simulink model "gnc_simplified"  (R2025b)
settings: Solver=ode2  StartTime=0.0  StopTime=inf  FixedStep=1/100  RelTol=1e-3
undefined symbols (not defined in the file or in its folder): DiscIntNeverNeededParam, dspblkCoreblockFVToolHelper, gcbh
libraries: simulink x5, eeGeneralControl x5
(part 1 of 4)
settings Model: Creator=ac112430  LastModifiedBy=ac124458
settings SolverCC: AlgebraicLoopSolver=TrustRegion
settings DataIOCC: ReturnWorkspaceOutputs=off
settings OptimizationCC: DefaultParameterBehavior=Inlined  DefaultUnderspecifiedDataType=single  PassReuseOutputArgsAs=Individual arguments  DifferentSizesBufferReuse=on  EfficientTunableParamExpr=on
settings DebuggingCC: ParameterPrecisionLossMsg=none  ParameterTunabilityLossMsg=error  UnconnectedInputMsg=warning  UnconnectedOutputMsg=warning  UnconnectedLineMsg=warning  BusObjectLabelMismatch=none  ArithmeticOperatorsInVariantConditions=warning
settings HardwareCC: ProdBitPerPointer=32.0  ProdBitPerSizeT=32.0  ProdBitPerPtrDiffT=32.0  ProdLargestAtomicInteger=Long  ProdLargestAtomicFloat=Double  ProdIntDivRoundTo=Undefined  ProdWordSize=32.0  ProdLongLongMode=on  ProdHWDeviceType=ARM Compatible->ARM Cortex
settings ModelReferenceCC: EnableRefExpFcnMdlSchedulingChecks=on  ModelReferenceNumInstancesAllowed=Single  PropagateSignalLabelsOutOfModel=off
settings SFSimCC: SimUseLocalCustomCode=off  MATLABDynamicMemAlloc=off  CustomCodeUndefinedFunction=UseInterfaceOnly
settings RTWCC: SystemTargetFile=ert.tlc  GenCodeOnly=on  TemplateMakefile=ert_default_tmf  RTWUseLocalCustomCode=off  IncludeHyperlinkInReport=on  GPUComputeCapability=3.5  Description=Embedded Coder
settings CodeAppCC: IgnoreCustomStorageClasses=off  MaxIdLength=2048.0  StateflowObjectComments=on
settings ERTTargetCC: ERTCustomFileTemplate=example_file_process.tlc  ConvertIfToSwitch=off  SuppressUnreachableDefaultCases=off  DynamicArrayContainerType=coder::array  TargetLangStandard=C99 (ISO)  GenerateSampleERTMain=on  SupportComplex=off  SupportVariableSizeSignals=on

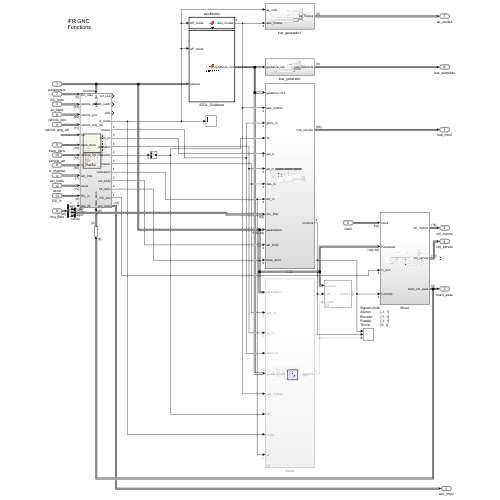
[thumbnail: Simulink's stored preview of the top-level diagram]
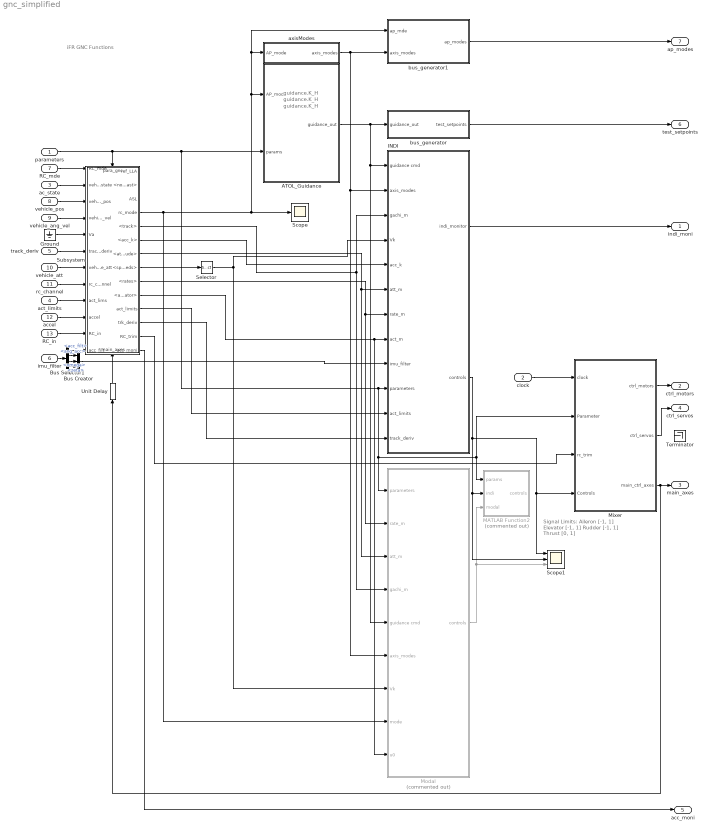
== system gnc_simplified ==
  note: iFR GNC Functions
  note: Signal Limits:
      | Aileron		[-1, 1]
      | Elevator		[-1, 1]
      | Rudder		[-1, 1]
      | Thrust		[0, 1]
  note: guidance.K_H
  note: guidance.K_H
  note: guidance.K_H
  note: guidance.K_H
  note: guidance.K_H
  parameters : Inport  OutDataTypeStr=Bus: IFRCG_Bus_Params_Gnc
  clock : Inport  Port=2  OutDataTypeStr=Bus: IFRCG_Bus_CodeGenInternalClock
  ac_state : Inport  Port=3  OutDataTypeStr=Bus: IFRCG_Bus_Topic_VehicleState  PortDimensions=1  SampleTime=[0.01,0]
  act_limits : Inport  Port=4  OutDataTypeStr=Bus: IFRCG_Bus_Topic_ActuatorLimits
  track_deriv : Inport  Port=5  OutDataTypeStr=Bus: IFRCG_Bus_Topic_TrackDerivMonitor
  imu_filter : Inport  Port=6  OutDataTypeStr=Bus: IFRCG_Bus_Topic_IfrImuFiltered
  RC_mde : Inport  Port=7  OutDataTypeStr=Bus: IFRCG_Bus_Topic_RcMode
  vehicle_pos : Inport  Port=8  OutDataTypeStr=Bus: IFRCG_Bus_Topic_VehicleLocalPosition
  vehicle_ang_vel : Inport  Port=9  OutDataTypeStr=Bus: IFRCG_Bus_Topic_VehicleAngularVelocity
  vehicle_att : Inport  Port=10  OutDataTypeStr=Bus: IFRCG_Bus_Topic_VehicleAttitude
  rc_channel : Inport  Port=11  OutDataTypeStr=Bus: IFRCG_Bus_Topic_RcChannels
  accel : Inport  Port=12  OutDataTypeStr=Bus: IFRCG_Bus_Topic_SensorAccel
  RC_in : Inport  Port=13  OutDataTypeStr=Bus: IFRCG_Bus_Topic_RcTrim
  ATOL_Guidance : MATLAB Function  TreatAsAtomicUnit=on
  Bus Creator : BusCreator  Inputs=3
  Bus Selector1 : BusSelector  OutputSignals=acc_filt,ang_acc,omega,zeta
  Ground : Ground
  INDI : Subsystem
  MATLAB Function2 : MATLAB Function  Commented=on  TreatAsAtomicUnit=on
  Mixer : Subsystem
  Modal : Subsystem  Commented=on
  Scope : Scope
      settings: DataLoggingVariableName=ScopeData4
  Scope1 : Scope  NumInputPorts=3
      settings: ActiveDisplayYMinimum=-1  ActiveDisplayYMaximum=1  DataLoggingVariableName=ScopeData2
  Selector : Selector  InputPortWidth=2  IndexOptions=Index vector (dialog)  Indices=1  OutputSizes=1
  Subsystem : Subsystem
      settings: PortSchema="{\"entries\":[{\"content\":{\"sides\":[{\"content\":{\"connectorIds\":[\"In1\",\"In2\",\"In3\",\"In4\",\"In5\",\"In6\",\"In7\",\"In8\",\"In9\",\"In10\",\"In11\",\"In12\"]},\"type\":\"ConnectorPlacement.EquallySpacedRectSide\",\"uuid\":\"eae11f8f-df23-443f-af8c-32e17e4605f0\"},{\"content\":{\"connectorIds\":[\"Out1\",\"Out2\",\"Out3\",\"Out4\",\"Out5\",\"Out6\",\"Out7\",\"Out8\",\"Out9\",\"Out10\",\"Out11\",\"Out12\",\"Out13\",\"Out14\"],\"side\":\"RIGHT\"},\"type\":\"ConnectorPlacement.EquallySpacedRectSide\",\"uuid\":\"25c6a971-14b0-4ed1-9e4e-a0a3a34e6a3d\"},{\"content\":{\"connectorIds\":[\"In13\"],\"side\":\"TOP\"},\"type\":\"ConnectorPlacement.EquallySpacedRectSide\",\"uuid\":\"38764348-8a10-4184-b281-810ae850f533\"},{\"content\":{\"connectorIds\":[\"In14\"],\"side\":\"BOTTOM\"},\"type\":\"ConnectorPlacement.EquallySpacedRectSide\",\"uuid\":\"a4d29612-f53e-4299-8f37-c5a613e7ffff\"}]},\"type\":\"ConnectorPlacement.EquallySpacedConnector\",\"uuid\":\"9dbe3133-1740-4116-b0d1-43b1503b7370\"}],\"packageUris\":[\"http://schema.mathworks.com/mf0/Connector/R2020b\"],\"version\":\"1.0\"}"
  Terminator : Terminator
  Unit Delay : UnitDelay  SampleTime=-1  HasFrameUpgradeWarning=on
  axisModes : MATLAB Function  TreatAsAtomicUnit=on
  bus_generator : Subsystem
  bus_generator1 : Subsystem
  indi_moni : Outport  OutDataTypeStr=Bus: IFRCG_Bus_Topic_IndiMonitor
  ctrl_motors : Outport  Port=2  OutDataTypeStr=Bus: IFRCG_Bus_Topic_ActuatorMotors  VectorParamsAs1DForOutWhenUnconnected=off
  main_axes : Outport  Port=3  OutDataTypeStr=Bus: IFRCG_Bus_Topic_MainCtrlAxes
  ctrl_servos : Outport  Port=4  OutDataTypeStr=Bus: IFRCG_Bus_Topic_ActuatorServos  VectorParamsAs1DForOutWhenUnconnected=off
  acc_moni : Outport  Port=5  OutDataTypeStr=Bus: IFRCG_Bus_Topic_AccelMonitor
  test_setpoints : Outport  Port=6  OutDataTypeStr=Bus: IFRCG_Bus_Topic_TestSetpointsMonitor
  ap_modes : Outport  Port=7  OutDataTypeStr=Bus: IFRCG_Bus_Topic_ApState
  wires:
  Mixer/1(ctrl_motors) -> ctrl_motors/1
  INDI/1(indi_monitor) -> indi_moni/1
  clock/1 -> Mixer/1(clock)
  ATOL_Guidance/1(guidance_out) -> Modal/5(guidance cmd), INDI/1(guidance cmd), bus_generator/1(guidance_out)
  Subsystem/8(<speeds>) -> Selector/1
  Selector/1 -> Modal/7(Vk), INDI/4(Vk)
  Subsystem/11(act_limits) -> INDI/11(act_limits)
  Subsystem/13(RC_trim) -> Mixer/3(rc_trim)
  Subsystem/6(<acc_k>) -> INDI/5(acc_k)
  Subsystem/7(<attitude>) -> Modal/3(att_m), INDI/6(att_m)
  Subsystem/5(<track>) -> INDI/3(gachi_m), Modal/4(gachi_m)
  ac_state/1 -> Subsystem/2(vehicle_state)
  Subsystem/9(<rates>) -> Modal/2(rate_m), INDI/7(rate_m)
  Subsystem/10(<actuator>) -> Modal/9(u0), INDI/8(act_m)
  Subsystem/12(trk_deriv) -> INDI/12(track_deriv)
  Modal/1(controls) -> Scope1/3, MATLAB Function2/3(modal)
  INDI/2(controls) -> Scope1/1, Mixer/4(Controls), Scope1/2, MATLAB Function2/2(indi)
  axisModes/1(axis_modes) -> Modal/6(axis_modes), INDI/2(axis_modes), bus_generator1/2(axis_modes)
  RC_mde/1 -> Subsystem/1(RC_mde)
  Mixer/3(main_ctrl_axes) -> Unit Delay/1, main_axes/1
  Mixer/2(ctrl_servos) -> ctrl_servos/1
  vehicle_ang_vel/1 -> Subsystem/4(vehicle_ang_vel)
  vehicle_att/1 -> Subsystem/7(vehicle_att)
  vehicle_pos/1 -> Subsystem/3(vehicle_pos)
  Ground/1 -> Subsystem/5(Va)
  act_limits/1 -> Subsystem/9(act_lims)
  Unit Delay/1 -> Subsystem/14(main_axes)
  rc_channel/1 -> Subsystem/8(rc_channel)
  accel/1 -> Subsystem/10(accel)
  imu_filter/1 -> Bus Selector1/1
  Bus Selector1/1 -> Subsystem/12(acc_filt)  "<acc_filt>"
  Bus Selector1/2 -> Bus Creator/1  "<ang_acc>"
  Bus Selector1/3 -> Bus Creator/2  "<omega>"
  Bus Selector1/4 -> Bus Creator/3  "<zeta>"
  Bus Creator/1 -> INDI/9(imu_filter)
  RC_in/1 -> Subsystem/11(RC_in)
  track_deriv/1 -> Subsystem/6(track_deriv)
  Subsystem/14(acc_moni) -> acc_moni/1
  Subsystem/4(rc_mode) -> bus_generator1/1(ap_mde), axisModes/1(AP_mode), ATOL_Guidance/1(AP_mode), Scope/1, Modal/8(mode)
  parameters/1 -> Subsystem/13(para_gnc), Modal/1(parameters), Mixer/2(Parameter), MATLAB Function2/1(params), INDI/10(parameters), ATOL_Guidance/2(params)
  bus_generator/1(test_setpoints) -> test_setpoints/1
  bus_generator1/1(ap_modes) -> ap_modes/1

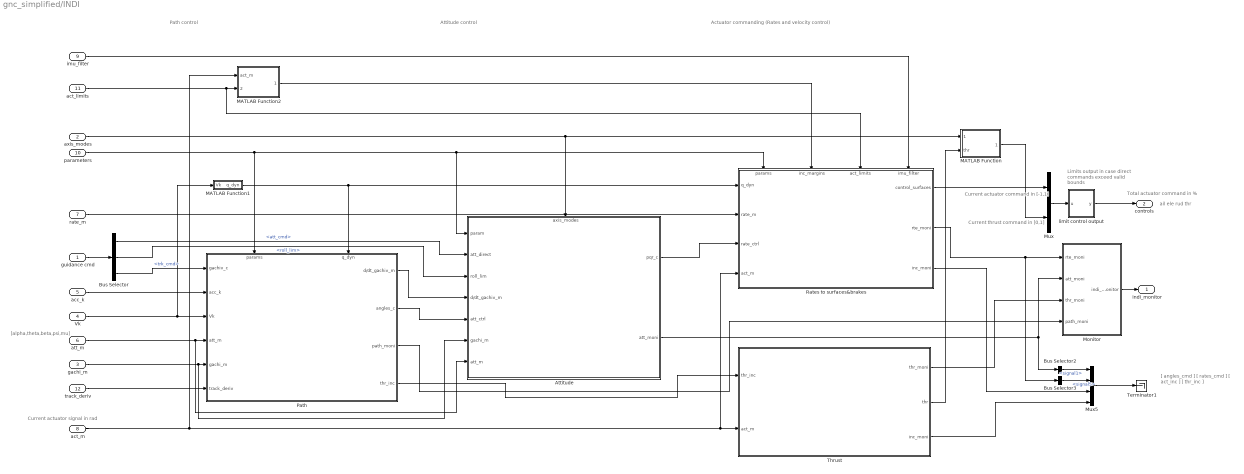
== system gnc_simplified/INDI ==
  note: [ angles_cmd	]
      | [ rates_cmd	]
      | [ act_inc		]
      | [ thr_inc		]
  note: ail ele rud thr
  note: Path control
  note: Current actuator
      | signal in rad
  note: [alpha,theta,beta,psi,mu]
  note: Attitude control
  note: Actuator commanding (Rates and velocity control)
  note: Limits output in case
      | direct commands
      | exceed valid bounds
  note: Current thrust command in [0,1]
  note: Total actuator
      | command in %
  note: Current actuator command in [-1,1]
  guidance cmd : Inport  OutDataTypeStr=Bus: IFRCG_Bus_GuidanceCmd
  axis_modes : Inport  Port=2  OutDataTypeStr=int8
  gachi_m : Inport  Port=3
  Vk : Inport  Port=4  PortDimensions=1
  acc_k : Inport  Port=5
  att_m : Inport  Port=6  OutDataTypeStr=single  PortDimensions=5
  rate_m : Inport  Port=7  OutDataTypeStr=single  PortDimensions=3
  act_m : Inport  Port=8  OutDataTypeStr=single  PortDimensions=4
  imu_filter : Inport  Port=9
  parameters : Inport  Port=10  OutDataTypeStr=Bus: IFRCG_Bus_Params_Gnc
  act_limits : Inport  Port=11
  track_deriv : Inport  Port=12  OutDataTypeStr=single  PortDimensions=2
  Attitude : Subsystem
      settings: PortSchema="{\"entries\":[{\"content\":{\"sides\":[{\"content\":{\"connectorIds\":[\"In1\",\"In2\",\"In3\",\"In4\",\"In5\",\"In6\",\"In7\"]},\"type\":\"ConnectorPlacement.EquallySpacedRectSide\",\"uuid\":\"b7c7e1a9-3024-403b-8101-4fc7eff0575e\"},{\"content\":{\"connectorIds\":[\"Out1\",\"Out2\"],\"side\":\"RIGHT\"},\"type\":\"ConnectorPlacement.EquallySpacedRectSide\",\"uuid\":\"cb53e122-7831-4c34-8aea-2b31ecc7af3b\"},{\"content\":{\"connectorIds\":[\"In8\"],\"side\":\"TOP\"},\"type\":\"ConnectorPlacement.EquallySpacedRectSide\",\"uuid\":\"4b53ef0a-efac-44dd-914a-4d2217d9826d\"}]},\"type\":\"ConnectorPlacement.EquallySpacedConnector\",\"uuid\":\"b88ec9b5-5f11-4970-871c-b4ff42b920b3\"}],\"packageUris\":[\"http://schema.mathworks.com/mf0/Connector/R2020b\"],\"version\":\"1.0\"}"
  Bus Selector : BusSelector  OutputSignals=att_cmd,roll_lim,trk_cmd
  Bus Selector2 : BusSelector  OutputSignals=signal1
  Bus Selector3 : BusSelector  OutputSignals=signal1.signal5
  MATLAB Function : MATLAB Function  TreatAsAtomicUnit=on
  MATLAB Function1 : MATLAB Function  TreatAsAtomicUnit=on
  MATLAB Function2 : MATLAB Function  TreatAsAtomicUnit=on
  Monitor : Subsystem
  Mux : Mux  Inputs=2
  Mux5 : Mux
  Path : Subsystem
      settings: PortSchema="{\"entries\":[{\"content\":{\"sides\":[{\"content\":{\"connectorIds\":[\"In1\",\"In2\",\"In3\",\"In4\",\"In5\",\"In6\"]},\"type\":\"ConnectorPlacement.EquallySpacedRectSide\",\"uuid\":\"aeeb4c65-4157-49e3-89f2-8442de4c35c3\"},{\"content\":{\"connectorIds\":[\"Out1\",\"Out2\",\"Out3\",\"Out4\"],\"side\":\"RIGHT\"},\"type\":\"ConnectorPlacement.EquallySpacedRectSide\",\"uuid\":\"9484377b-093c-4072-8beb-471d4a7ab8a9\"},{\"content\":{\"connectorIds\":[\"In7\",\"In8\"],\"side\":\"TOP\"},\"type\":\"ConnectorPlacement.EquallySpacedRectSide\",\"uuid\":\"c6253d73-40c9-4522-8e2e-6cc388a7bc53\"},{\"content\":{\"side\":\"BOTTOM\"},\"type\":\"ConnectorPlacement.EquallySpacedRectSide\",\"uuid\":\"b5f53673-25a9-4222-bcda-17be59006191\"}]},\"type\":\"ConnectorPlacement.EquallySpacedConnector\",\"uuid\":\"6ddcfaaa-ad15-4bea-bdab-3495e7fd8cf9\"}],\"packageUris\":[\"http://schema.mathworks.com/mf0/Connector/R2020b\"],\"version\":\"1.0\"}"
  Rates to surfaces&brakes : Subsystem
      settings: PortSchema="{\"entries\":[{\"content\":{\"sides\":[{\"content\":{\"connectorIds\":[\"In1\",\"In2\",\"In3\",\"In4\"]},\"type\":\"ConnectorPlacement.EquallySpacedRectSide\",\"uuid\":\"38e84281-7140-4c55-a86a-c71fe3b9f0d7\"},{\"content\":{\"connectorIds\":[\"Out1\",\"Out2\",\"Out3\"],\"side\":\"RIGHT\"},\"type\":\"ConnectorPlacement.EquallySpacedRectSide\",\"uuid\":\"18979a8d-3905-4a49-86c3-949277d06de1\"},{\"content\":{\"connectorIds\":[\"In5\",\"In6\",\"In7\",\"In8\"],\"side\":\"TOP\"},\"type\":\"ConnectorPlacement.EquallySpacedRectSide\",\"uuid\":\"2ae550e8-8587-46c8-a90f-db3ecfdcb8e8\"},{\"content\":{\"side\":\"BOTTOM\"},\"type\":\"ConnectorPlacement.EquallySpacedRectSide\",\"uuid\":\"d561a624-fdf7-40a1-bac0-8ec2b91f5f36\"}]},\"type\":\"ConnectorPlacement.EquallySpacedConnector\",\"uuid\":\"df4b2bf7-ea7e-4f09-bf8e-e1a831543136\"}],\"packageUris\":[\"http://schema.mathworks.com/mf0/Connector/R2020b\"],\"version\":\"1.0\"}"
  Terminator1 : Terminator
  Thrust : Subsystem
  limit control output : MATLAB Function  TreatAsAtomicUnit=on
  indi_monitor : Outport  OutDataTypeStr=Bus: IFRCG_Bus_Topic_IndiMonitor
  controls : Outport  Port=2  OutDataTypeStr=single  PortDimensions=4  VectorParamsAs1DForOutWhenUnconnected=off
  wires:
  Bus Selector/2 -> Attitude/3(roll_lim)  "<roll_lim>"
  Thrust/3(inc_moni) -> Mux5/4
  Path/3(path_moni) -> Monitor/4(path_moni)
  Rates to surfaces&brakes/3(inc_moni) -> Mux5/3
  parameters/1 -> Rates to surfaces&brakes/5(params), Attitude/1(param), Path/7(params)
  Mux5/1 -> Terminator1/1
  att_m/1 -> Attitude/7(att_m), Path/4(att_m)
  acc_k/1 -> Path/2(acc_k)
  Rates to surfaces&brakes/1(control_surfaces) -> Mux/1
  Bus Selector/3 -> Path/1(gachiv_c)  "<trk_cmd>"
  Attitude/1(pqr_c) -> Rates to surfaces&brakes/3(rate_ctrl)
  Vk/1 -> MATLAB Function1/1(Vk), Path/3(Vk)
  act_m/1 -> Thrust/2(act_m), Rates to surfaces&brakes/4(act_m), MATLAB Function2/1(act_m)
  Path/4(thr_inc) -> Thrust/1(thr_inc)
  rate_m/1 -> Rates to surfaces&brakes/2(rate_m)
  Path/2(angles_c) -> Attitude/5(att_ctrl)
  Thrust/2(thr) -> MATLAB Function/2(thr)
  guidance cmd/1 -> Bus Selector/1
  Path/1(d/dt_gachiv_m) -> Attitude/4(d/dt_gachiv_m)
  Thrust/1(thr_moni) -> Monitor/3(thr_moni)
  Rates to surfaces&brakes/2(rte_moni) -> Monitor/1(rte_moni), Bus Selector3/1
  gachi_m/1 -> Attitude/6(gachi_m), Path/5(gachi_m)
  Monitor/1(indi_monitor) -> indi_monitor/1
  Bus Selector2/1 -> Mux5/1  "<signal1>"
  Bus Selector3/1 -> Mux5/2  "<signal5>"
  Attitude/2(att_moni) -> Monitor/2(att_moni), Bus Selector2/1
  track_deriv/1 -> Path/6(track_deriv)
  limit control output/1(y) -> controls/1
  act_limits/1 -> Rates to surfaces&brakes/7(act_limits), MATLAB Function2/2(act_limit)
  MATLAB Function2/1(inc_margins) -> Rates to surfaces&brakes/6(inc_margins)
  imu_filter/1 -> Rates to surfaces&brakes/8(imu_filter)
  Mux/1 -> limit control output/1(u)
  axis_modes/1 -> MATLAB Function/1(axis_modes), Attitude/8(axis_modes)
  MATLAB Function/1(thr_cmd) -> Mux/2
  Bus Selector/1 -> Attitude/2(att_direct)  "<att_cmd>"
  MATLAB Function1/1(q_dyn) -> Rates to surfaces&brakes/1(q_dyn), Path/8(q_dyn)

== system gnc_simplified/Mixer ==
  note: control allocation for elevator and rudder
  note: Reversing ap output according to servo mounting direction;
  note: Adjusting output
      | according to servo
      | limitations
  note: Sorting for channel
      | scaling in Pixhawk
  note: thr
      | ail
      | ele
      | rud
  note: Output for Gram:
      | 1 Thrust
      | 2 Aileron right
      | 3 Aileron left
      | 4 Flaperon right
      | 5 Flaperon left
      | 6 Elevator/Rudder right
      | 7 Elevator/Rudder left
      | 8 Gear
      | 9 Safety
      | 10 Arming
      | 11 Mode switch
  note: Signal Limits:
      | Aileron		[-1, 1]
      | Elevator		[-1, 1]
      | Rudder		[-1, 1]
      | Thrust		[0, 1]
  note: Signal Limits:
      | Aileron		[-1, 1]
      | Elevator		[-1, 1]
      | Rudder		[-1, 1]
      | Thrust		[0, 1]
  clock : Inport  OutDataTypeStr=Bus: IFRCG_Bus_CodeGenInternalClock
  Parameter : Inport  Port=2  OutDataTypeStr=Bus: IFRCG_Bus_Params_Gnc
  rc_trim : Inport  Port=3
  Controls : Inport  Port=4  OutDataTypeStr=single  PortDimensions=4
  Bus Selector : BusSelector  OutputSignals=sys_time_us
  Constant2 : Constant  Value=zeros(8,1)  OutDataTypeStr=single
  Data Type Conversion1 : DataTypeConversion  OutDataTypeStr=uint64  SaturateOnIntegerOverflow=off  RndMeth=Floor
  MATLAB Function1 : MATLAB Function  TreatAsAtomicUnit=on
  MATLAB Function2 : MATLAB Function  TreatAsAtomicUnit=on
  PWM Limiter : MATLAB Function  TreatAsAtomicUnit=on
  Scope1 : Scope  NumInputPorts=2
      settings: ActiveDisplayYMinimum=-1.25  ActiveDisplayYMaximum=1.25  DataLoggingVariableName=ScopeData8
  Scope2 : Scope
      settings: ActiveDisplayYMinimum=-2.2855338454246521  ActiveDisplayYMaximum=2.2855338454246521  DataLoggingVariableName=ScopeData2
  Selector1 : Selector  InputPortWidth=4  IndexOptions=Index vector (dialog)  Indices=[4 1 2 3]  OutputSizes=1
  Terminator : Terminator
  _bus_creator1 : Subsystem
  _bus_creator2 : Subsystem  Commented=on
  bus_generator : Subsystem
  scale_RC_thr : MATLAB Function  TreatAsAtomicUnit=on
  scale_thr : MATLAB Function  TreatAsAtomicUnit=on
  ctrl_motors : Outport  OutDataTypeStr=Bus: IFRCG_Bus_Topic_ActuatorMotors  VectorParamsAs1DForOutWhenUnconnected=off
  ctrl_servos : Outport  Port=2  OutDataTypeStr=Bus: IFRCG_Bus_Topic_ActuatorServos  VectorParamsAs1DForOutWhenUnconnected=off
  main_ctrl_axes : Outport  Port=3  OutDataTypeStr=Bus: IFRCG_Bus_Topic_MainCtrlAxes
  wires:
  Controls/1 -> scale_thr/1(in)  "ail ele rud thr nw"
  Parameter/1 -> PWM Limiter/1(parameter), MATLAB Function1/1(params)
  clock/1 -> Bus Selector/1
  rc_trim/1 -> scale_RC_thr/1(in)
  _bus_creator2/1(actuator_controls) -> Terminator/1
  Constant2/1 -> _bus_creator2/1(control)
  scale_RC_thr/1(out) -> MATLAB Function1/3(rc_controls)
  Selector1/1 -> bus_generator/1(In1), Scope1/2, MATLAB Function2/1(controls_in)
  scale_thr/1(out) -> MATLAB Function1/2(ap_controls), Scope1/1
  MATLAB Function2/1(controls_out) -> PWM Limiter/2(controls)
  _bus_creator1/2(ctrl_servos) -> ctrl_servos/1
  bus_generator/1(main_ctrl_axes) -> main_ctrl_axes/1
  PWM Limiter/1(controlsLtd) -> _bus_creator1/1(control), Scope2/1
  Data Type Conversion1/1 -> _bus_creator1/2(timestamp_sample)
  Bus Selector/1 -> Data Type Conversion1/1, _bus_creator2/2(timestamp_sample)  "<sys_time_us>"
  _bus_creator1/1(ctrl_motors) -> ctrl_motors/1
  MATLAB Function1/1(controls) -> Selector1/1

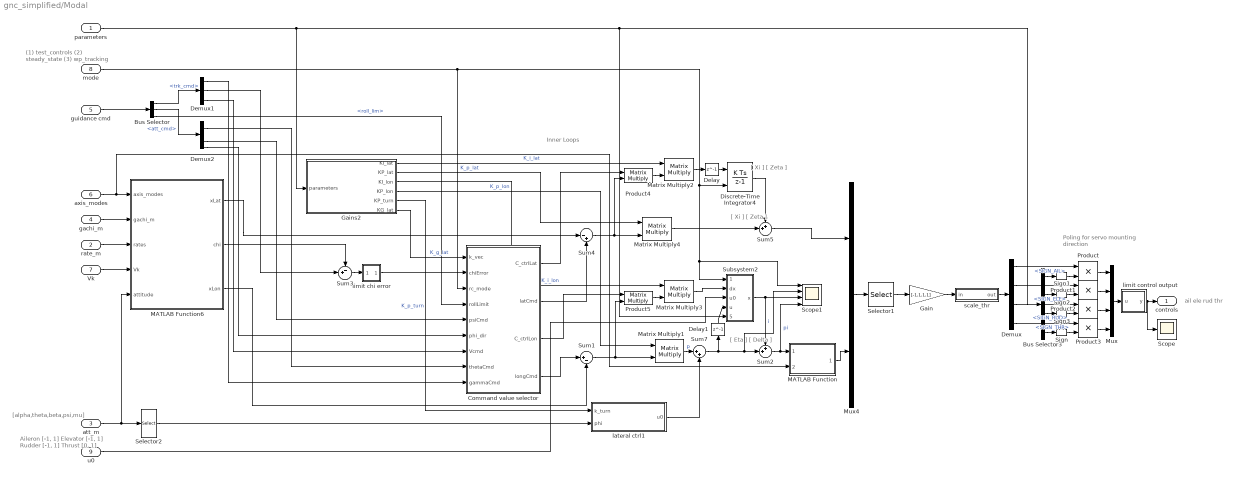
== system gnc_simplified/Modal ==
  note: [alpha,theta,beta,psi,mu]
  note: ail ele rud thr
  note: Poling for servo
      | mounting direction
  note: [ Xi     ]
      | [ Zeta ]
  note: Inner Loops
  note: [ Xi     ]
      | [ Zeta ]
  note: [ Eta    ]
      | [ Delta ]
  note: (1) test_controls
      | (2) steady_state
      | (3) wp_tracking
  note: Aileron		[-1, 1]
      | Elevator		[-1, 1]
      | Rudder		[-1, 1]
      | Thrust		[0, 1]
  parameters : Inport  OutDataTypeStr=Bus: IFRCG_Bus_Params_Gnc
  rate_m : Inport  Port=2  OutDataTypeStr=single  PortDimensions=3
  att_m : Inport  Port=3  OutDataTypeStr=single  PortDimensions=5
  gachi_m : Inport  Port=4
  guidance cmd : Inport  Port=5  OutDataTypeStr=Bus: IFRCG_Bus_GuidanceCmd
  axis_modes : Inport  Port=6
  Vk : Inport  Port=7  PortDimensions=1
  mode : Inport  Port=8  OutDataTypeStr=uint8
  u0 : Inport  Port=9  OutDataTypeStr=single  PortDimensions=4
  Bus Selector : BusSelector  OutputSignals=trk_cmd,att_cmd,roll_lim
  Bus Selector3 : BusSelector  OutputSignals=Ifr_Gnc.SIGN_AIL,Ifr_Gnc.SIGN_ELE,Ifr_Gnc.SIGN_RUD,Ifr_Gnc.SIGN_THR
  Command value selector : MATLAB Function  TreatAsAtomicUnit=on
  Delay : Delay  DelayLength=1
  Delay1 : Delay  DelayLength=1
  Demux : Demux
  Demux1 : Demux  Outputs=3
  Demux2 : Demux  Outputs=5
  Discrete-Time Integrator4 : DiscreteIntegrator  ExternalReset=either  SampleTime=-1  LimitOutput=on  UpperSaturationLimit=15  LowerSaturationLimit=-15  ICPrevOutput=DiscIntNeverNeededParam  ICPrevScaledInput=DiscIntNeverNeededParam
  Gain : Gain  Gain=[-1,1,1,1]
  Gains2 : MATLAB Function  TreatAsAtomicUnit=on
  MATLAB Function : MATLAB Function  TreatAsAtomicUnit=on
  MATLAB Function6 : MATLAB Function  TreatAsAtomicUnit=on
  Matrix Multiply{1..4} (4 alike) : Product  Multiplication=Matrix(*)
  Mux : Mux
  Mux4 : Mux  Inputs=2
  Product{,1..3} (4 alike) : Product  OutDataTypeStr=single
  Product4 : Product  Multiplication=Matrix(*)
  Product5 : Product  Multiplication=Matrix(*)
  Scope : Scope
      settings: DataLoggingVariableName=ScopeData9
  Scope1 : Scope  NumInputPorts=4
      settings: DataLoggingVariableName=ScopeData10
  Selector1 : Selector  InputPortWidth=4  IndexOptions=Index vector (dialog)  Indices=[1,3,2,4]  OutputSizes=1
  Selector2 : Selector  InputPortWidth=5  IndexOptions=Index vector (dialog)  Indices=5  OutputSizes=1
  Sign{,1..3} (4 alike) : Signum
  Subsystem2 : Subsystem
      mask Display:
      | disp('\bf\fontsize{12}\int dx', 'texmode', 'on')
      | port_label('input', 2, 'dx', 'texmode', 'on')
      | port_label('input', 1, 'Tr')
      | port_label('input', 3, 'u_0', 'texmode', 'on')
      | port_label('input', 4, 'u_P', 'texmode', 'on')
      | 
      | port_label('output', 1, 'x', 'texmode', 'on')
  Sum1 : Sum  Inputs=|+-
  Sum2 : Sum  Inputs=++|
  Sum3 : Sum  Inputs=-+|
  Sum4 : Sum  Inputs=|-+
  Sum5 : Sum  Inputs=++|
  Sum7 : Sum  Inputs=|++
  lateral ctrl1 : MATLAB Function  TreatAsAtomicUnit=on
  limit chi error : MATLAB Function  TreatAsAtomicUnit=on
  limit control output : MATLAB Function  TreatAsAtomicUnit=on
  scale_thr : MATLAB Function  TreatAsAtomicUnit=on
  controls : Outport  OutDataTypeStr=single  PortDimensions=4  VectorParamsAs1DForOutWhenUnconnected=off
  wires:
  limit control output/1(y) -> Scope/1, controls/1
  guidance cmd/1 -> Bus Selector/1
  Gain/1 -> scale_thr/1(in)
  Mux4/1 -> Selector1/1
  Selector1/1 -> Gain/1
  Bus Selector/1 -> Demux1/1  "<trk_cmd>"
  Demux/4 -> Product3/1
  Demux/2 -> Product1/1
  Bus Selector3/3 -> Sign3/1  "<SIGN_RUD>"
  Sign/1 -> Product3/2
  Bus Selector3/1 -> Sign1/1  "<SIGN_AIL>"
  Demux/1 -> Product/1
  Bus Selector3/2 -> Sign2/1  "<SIGN_ELE>"
  Sign1/1 -> Product/2
  Demux/3 -> Product2/1
  Bus Selector3/4 -> Sign/1  "<SIGN_THR>"
  Sign2/1 -> Product1/2
  Sign3/1 -> Product2/2
  Product/1 -> Mux/1
  Product1/1 -> Mux/2
  Product2/1 -> Mux/3
  Product3/1 -> Mux/4
  Mux/1 -> limit control output/1(u)
  scale_thr/1(out) -> Demux/1
  MATLAB Function/1(ele_thr_cmd) -> Mux4/2
  Bus Selector/2 -> Demux2/1  "<att_cmd>"
  parameters/1 -> Gains2/1(parameters), Bus Selector3/1, Subsystem2/5(param)
  Sum5/1 -> Mux4/1
  Delay1/1 -> Subsystem2/4(u)
  Delay/1 -> Discrete-Time Integrator4/1
  Command value selector/1(C_ctrlLat) -> Product4/1
  Demux2/4 -> Command value selector/5(psiCmd)
  Gains2/5(KP_turn) -> lateral ctrl1/1(k_turn)  "K_p_turn"
  Product4/1 -> Matrix Multiply2/2
  Gains2/1(KI_lat) -> Matrix Multiply2/1  "K_i_lat"
  Gains2/3(KI_lon) -> Matrix Multiply3/1  "K_i_lon"
  Matrix Multiply1/1 -> Sum7/1  "p"
  Command value selector/2(latCmd) -> Sum4/2
  Gains2/2(KP_lat) -> Matrix Multiply4/1  "K_p_lat"
  Demux1/3 -> Command value selector/7(Vcmd)
  limit chi error/1(y) -> Command value selector/2(chiError)
  Product5/1 -> Matrix Multiply3/2
  Command value selector/4(longCmd) -> Sum1/1
  Demux2/2 -> Command value selector/8(thetaCmd)
  Matrix Multiply3/1 -> Subsystem2/2(dx)
  Command value selector/3(C_ctrlLon) -> Product5/1
  Discrete-Time Integrator4/1 -> Sum5/1
  Demux1/1 -> Command value selector/9(gammaCmd)
  Gains2/4(KP_lon) -> Matrix Multiply1/1  "K_p_lon"
  Subsystem2/1(x) -> Sum2/1, Scope1/3  "i"
  Matrix Multiply2/1 -> Delay/1
  MATLAB Function6/3(xLon) -> Sum1/2
  Sum4/1 -> Product4/2, Matrix Multiply4/2
  lateral ctrl1/1(u0) -> Sum7/2
  MATLAB Function6/1(xLat) -> Sum4/1
  Sum2/1 -> Scope1/4, MATLAB Function/1(ele_thr)  "pi"
  Selector2/1 -> lateral ctrl1/2(phi)
  Bus Selector/3 -> Command value selector/4(rollLimit)  "<roll_lim>"
  u0/1 -> Subsystem2/3(u0)
  Sum3/1 -> limit chi error/1(u)
  Sum1/1 -> Product5/2, Matrix Multiply1/2
  mode/1 -> Discrete-Time Integrator4/2, Scope1/1, Subsystem2/1(mode), Command value selector/3(rc_mode)
  Sum7/1 -> Delay1/1, Scope1/2, Sum2/2
  Matrix Multiply4/1 -> Sum5/2
  MATLAB Function6/2(chi) -> Sum3/1
  att_m/1 -> MATLAB Function6/5(attitude), Selector2/1
  Vk/1 -> MATLAB Function6/4(Vk)
  gachi_m/1 -> MATLAB Function6/2(gachi_m)
  rate_m/1 -> MATLAB Function6/3(rates)
  Demux1/2 -> Sum3/2
  Demux2/5 -> Command value selector/6(phi_dir)
  Gains2/6(KG_lat) -> Command value selector/1(k_vec)  "K_g_lat"
  axis_modes/1 -> MATLAB Function/2(axis_modes), MATLAB Function6/1(axis_modes)

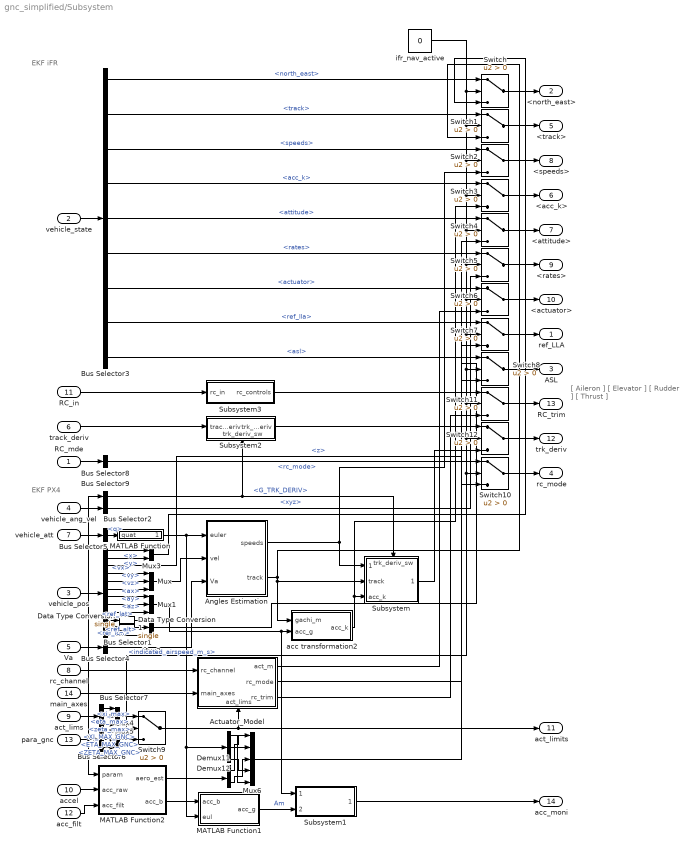
== system gnc_simplified/Subsystem ==
  note: EKF iFR
  note: EKF PX4
  note: [ Aileron	  ]
      | [ Elevator ]
      | [ Rudder	  ]
      | [ Thrust	  ]
  RC_mde : Inport  OutDataTypeStr=Bus: IFRCG_Bus_Topic_RcMode
  vehicle_state : Inport  Port=2  OutDataTypeStr=Bus: IFRCG_Bus_Topic_VehicleState
  vehicle_pos : Inport  Port=3  OutDataTypeStr=Bus: IFRCG_Bus_Topic_VehicleLocalPosition
  vehicle_ang_vel : Inport  Port=4  OutDataTypeStr=Bus: IFRCG_Bus_Topic_VehicleAngularVelocity
  Va : Inport  Port=5  OutDataTypeStr=Bus: IFRCG_Bus_Topic_Airspeed
  track_deriv : Inport  Port=6  OutDataTypeStr=Bus: IFRCG_Bus_Topic_TrackDerivMonitor
  vehicle_att : Inport  Port=7  OutDataTypeStr=Bus: IFRCG_Bus_Topic_VehicleAttitude
  rc_channel : Inport  Port=8  OutDataTypeStr=Bus: IFRCG_Bus_Topic_RcChannels
  act_lims : Inport  Port=9  OutDataTypeStr=Bus: IFRCG_Bus_Topic_ActuatorLimits
  accel : Inport  Port=10  OutDataTypeStr=Bus: IFRCG_Bus_Topic_SensorAccel
  RC_in : Inport  Port=11  OutDataTypeStr=Bus: IFRCG_Bus_Topic_RcTrim
  acc_filt : Inport  Port=12
  para_gnc : Inport  Port=13  OutDataTypeStr=Bus: IFRCG_Bus_Params_Gnc
  main_axes : Inport  Port=14  OutDataTypeStr=Bus: IFRCG_Bus_Topic_MainCtrlAxes
  Actuator_Model : Subsystem
      settings: PortSchema="{\"entries\":[{\"content\":{\"sides\":[{\"content\":{\"connectorIds\":[\"In1\",\"In2\"]},\"type\":\"ConnectorPlacement.EquallySpacedRectSide\",\"uuid\":\"0b560cb0-425b-4e75-ad69-9f3dd2ae247d\"},{\"content\":{\"connectorIds\":[\"Out1\",\"Out2\",\"Out3\"],\"side\":\"RIGHT\"},\"type\":\"ConnectorPlacement.EquallySpacedRectSide\",\"uuid\":\"67043da2-be34-4466-be37-15cebe548400\"},{\"content\":{\"side\":\"TOP\"},\"type\":\"ConnectorPlacement.EquallySpacedRectSide\",\"uuid\":\"dbc9e13d-738a-4a6f-867f-431ba88297cf\"},{\"content\":{\"connectorIds\":[\"In3\"],\"side\":\"BOTTOM\"},\"type\":\"ConnectorPlacement.EquallySpacedRectSide\",\"uuid\":\"14b82ace-20eb-4480-853b-ffa5dbbc5ee0\"}]},\"type\":\"ConnectorPlacement.EquallySpacedConnector\",\"uuid\":\"43045ae4-5565-43c8-8df8-998e069be6cd\"}],\"packageUris\":[\"http://schema.mathworks.com/mf0/Connector/R2020b\"],\"version\":\"1.0\"}"
  Angles Estimation : MATLAB Function  TreatAsAtomicUnit=on
  Bus Selector1 : BusSelector  OutputSignals=x,y,z,vx,vy,vz,ax,ay,az,ref_lat,ref_lon,ref_alt
  Bus Selector2 : BusSelector  OutputSignals=xyz
  Bus Selector3 : BusSelector  OutputSignals=north_east,track,speeds,acc_k,attitude,rates,actuator,ref_lla,asl
  Bus Selector4 : BusSelector  OutputSignals=indicated_airspeed_m_s
  Bus Selector5 : BusSelector  OutputSignals=q
  Bus Selector6 : BusSelector  OutputSignals=Ifr_Gnc.XI_MAX_GNC,Ifr_Gnc.ETA_MAX_GNC,Ifr_Gnc.ZETA_MAX_GNC
  Bus Selector7 : BusSelector  OutputSignals=xi_max,eta_max,zeta_max
  Bus Selector8 : BusSelector  OutputSignals=rc_mode
  Bus Selector9 : BusSelector  OutputSignals=Ifr_Gnc.G_TRK_DERIV
  Data Type Conversion : DataTypeConversion  OutDataTypeStr=single  SaturateOnIntegerOverflow=off  RndMeth=Floor
  Data Type Conversion1 : DataTypeConversion  OutDataTypeStr=single  SaturateOnIntegerOverflow=off  RndMeth=Floor
  Demux11 : Demux  Outputs=2
  Demux12 : Demux  Outputs=3
  MATLAB Function : MATLAB Function  TreatAsAtomicUnit=on
  MATLAB Function1 : MATLAB Function  TreatAsAtomicUnit=on
  MATLAB Function2 : MATLAB Function  TreatAsAtomicUnit=on
  Mux{,1..2,4..5} (5 alike) : Mux  Inputs=3
  Mux3 : Mux  Inputs=2
  Mux6 : Mux  Inputs=5
  Subsystem : Subsystem
      settings: PortSchema="{\"entries\":[{\"content\":{\"sides\":[{\"content\":{\"connectorIds\":[\"In1\",\"In2\",\"In3\"]},\"type\":\"ConnectorPlacement.EquallySpacedRectSide\",\"uuid\":\"d3f70b0d-5808-41a1-901a-3e2b7a37eb93\"},{\"content\":{\"connectorIds\":[\"Out1\"],\"side\":\"RIGHT\"},\"type\":\"ConnectorPlacement.EquallySpacedRectSide\",\"uuid\":\"dc4ca20c-eb1b-4454-88d2-269a48f937e4\"},{\"content\":{\"connectorIds\":[\"In4\"],\"side\":\"TOP\"},\"type\":\"ConnectorPlacement.EquallySpacedRectSide\",\"uuid\":\"1dace743-43be-4004-9081-e38a97e7a582\"}]},\"type\":\"ConnectorPlacement.EquallySpacedConnector\",\"uuid\":\"5771c896-d5ee-401f-a70a-0ba475a64d58\"}],\"packageUris\":[\"http://schema.mathworks.com/mf0/Connector/R2020b\"],\"version\":\"1.0\"}"
  Subsystem1 : Subsystem
  Subsystem2 : Subsystem
      settings: PortSchema="{\"entries\":[{\"content\":{\"sides\":[{\"content\":{\"connectorIds\":[\"In1\"]},\"type\":\"ConnectorPlacement.EquallySpacedRectSide\",\"uuid\":\"c249bde2-4580-435b-8669-29d5f206d176\"},{\"content\":{\"connectorIds\":[\"Out1\"],\"side\":\"RIGHT\"},\"type\":\"ConnectorPlacement.EquallySpacedRectSide\",\"uuid\":\"60962190-2f64-42e9-bf1a-6d4a20eea6b3\"},{\"content\":{\"side\":\"TOP\"},\"type\":\"ConnectorPlacement.EquallySpacedRectSide\",\"uuid\":\"d4f64458-133b-4324-95a6-14c38555dd9a\"},{\"content\":{\"connectorIds\":[\"In2\"],\"side\":\"BOTTOM\"},\"type\":\"ConnectorPlacement.EquallySpacedRectSide\",\"uuid\":\"5ed7f531-edd6-4543-875a-2dd5af02d360\"}]},\"type\":\"ConnectorPlacement.EquallySpacedConnector\",\"uuid\":\"8eaaea99-2870-4f7f-ab6c-9598fb8c4fc7\"}],\"packageUris\":[\"http://schema.mathworks.com/mf0/Connector/R2020b\"],\"version\":\"1.0\"}"
  Subsystem3 : Subsystem
  Switch{,1..12} (13 alike) : Switch  Criteria=u2 > Threshold  SaturateOnIntegerOverflow=off  InputSameDT=off
  acc transformation2 : MATLAB Function  TreatAsAtomicUnit=on
  ifr_nav_active : Constant  Value=0
  ref_LLA : Outport
  <north_east> : Outport  Port=2
  ASL : Outport  Port=3
  rc_mode : Outport  Port=4  OutDataTypeStr=uint8  PortDimensions=1
  <track> : Outport  Port=5
  <acc_k> : Outport  Port=6
  <attitude> : Outport  Port=7
  <speeds> : Outport  Port=8
  <rates> : Outport  Port=9
  <actuator> : Outport  Port=10
  act_limits : Outport  Port=11
  trk_deriv : Outport  Port=12  PortDimensions=2
  RC_trim : Outport  Port=13  PortDimensions=4
  acc_moni : Outport  Port=14  OutDataTypeStr=Bus: IFRCG_Bus_Topic_AccelMonitor
  wires:
  Bus Selector3/5 -> Switch4/1  "<attitude>"
  Bus Selector3/4 -> Switch3/1  "<acc_k>"
  Bus Selector3/7 -> Switch6/1  "<actuator>"
  Bus Selector3/1 -> Switch/1  "<north_east>"
  Bus Selector3/2 -> Switch1/1  "<track>"
  Bus Selector3/6 -> Switch5/1  "<rates>"
  Bus Selector3/3 -> Switch2/1  "<speeds>"
  vehicle_state/1 -> Bus Selector3/1
  Bus Selector2/1 -> Switch5/3  "<xyz>"
  Angles Estimation/2(track) -> Subsystem/2(track), acc transformation2/1(gachi_m), Switch1/3
  vehicle_att/1 -> Bus Selector5/1
  Bus Selector5/1 -> MATLAB Function/1(quat)  "<q>"
  Bus Selector1/2 -> Mux3/2  "<y>"
  vehicle_ang_vel/1 -> Bus Selector2/1
  Bus Selector4/1 -> Angles Estimation/3(Va)  "<indicated_airspeed_m_s>"
  Bus Selector1/5 -> Mux/2  "<vy>"
  Va/1 -> Bus Selector4/1
  Bus Selector1/4 -> Mux/1  "<vx>"
  vehicle_pos/1 -> Bus Selector1/1
  Bus Selector1/6 -> Mux/3  "<vz>"
  Mux/1 -> Angles Estimation/2(vel)
  Bus Selector1/1 -> Mux3/1  "<x>"
  Bus Selector1/7 -> Mux1/1  "<ax>"
  Bus Selector1/8 -> Mux1/2  "<ay>"
  Bus Selector1/9 -> Mux1/3  "<az>"
  Mux1/1 -> Subsystem1/1(acc_g_vlp), acc transformation2/2(acc_g)
  acc transformation2/1(acc_k) -> Switch3/3, Subsystem/3(acc_k)
  MATLAB Function/1(eul_rad) -> Angles Estimation/1(euler), MATLAB Function1/2(eul), Demux12/1
  Angles Estimation/1(speeds) -> Subsystem/1(speeds), Switch2/3
  Mux3/1 -> Switch/3
  Bus Selector3/8 -> Switch7/1  "<ref_lla>"
  Bus Selector3/9 -> Switch8/1  "<asl>"
  Switch/1 -> <north_east>/1
  Switch1/1 -> <track>/1
  Switch2/1 -> <speeds>/1
  Switch3/1 -> <acc_k>/1
  Switch4/1 -> <attitude>/1
  Switch5/1 -> <rates>/1
  Switch8/1 -> ASL/1
  Switch6/1 -> <actuator>/1
  Switch7/1 -> ref_LLA/1
  Actuator_Model/1(act_m) -> Switch6/3
  Bus Selector1/10 -> Data Type Conversion/1  "<ref_lat>"
  Bus Selector1/11 -> Data Type Conversion1/1  "<ref_lon>"
  Bus Selector1/12 -> Mux2/3  "<ref_alt>"
  Bus Selector1/3 -> Switch8/3  "<z>"
  rc_channel/1 -> Actuator_Model/1(rc_channel)
  main_axes/1 -> Actuator_Model/2(main_axes)
  act_lims/1 -> Bus Selector7/1
  Switch9/1 -> Actuator_Model/3(act_lims), act_limits/1
  ifr_nav_active/1 -> Switch/2, Switch1/2, Switch2/2, Switch3/2, Switch4/2, Switch5/2, Switch6/2, Switch7/2, Switch11/2, Switch12/2, Switch9/2, Switch10/2, Switch8/2
  para_gnc/1 -> MATLAB Function2/1(param), Bus Selector9/1, Bus Selector6/1
  Mux4/1 -> Switch9/3
  Bus Selector6/1 -> Mux4/1  "<XI_MAX_GNC>"
  Bus Selector6/2 -> Mux4/2  "<ETA_MAX_GNC>"
  Bus Selector6/3 -> Mux4/3  "<ZETA_MAX_GNC>"
  Bus Selector7/1 -> Mux5/1  "<xi_max>"
  Bus Selector7/2 -> Mux5/2  "<eta_max>"
  Bus Selector7/3 -> Mux5/3  "<zeta_max>"
  Mux5/1 -> Switch9/1
  Actuator_Model/2(rc_mode) -> Switch10/3
  RC_mde/1 -> Bus Selector8/1
  Switch10/1 -> rc_mode/1
  Demux12/1 -> Mux6/5
  Demux11/2 -> Mux6/3
  Demux11/1 -> Mux6/1
  Demux12/3 -> Mux6/4
  Demux12/2 -> Mux6/2
  Mux6/1 -> Switch4/3
  MATLAB Function2/1(aero_est) -> Demux11/1
  accel/1 -> MATLAB Function2/2(acc_raw)
  acc_filt/1 -> MATLAB Function2/3(acc_filt)
  Bus Selector8/1 -> Switch10/1  "<rc_mode>"
  Mux2/1 -> Switch7/3
  Data Type Conversion/1 -> Mux2/1
  Data Type Conversion1/1 -> Mux2/2
  Actuator_Model/3(rc_trim) -> Switch11/3
  Switch11/1 -> RC_trim/1
  Subsystem3/1(rc_controls) -> Switch11/1
  Switch12/1 -> trk_deriv/1
  Subsystem2/1(trk_deriv) -> Switch12/1
  Subsystem/1(d_trk_moni) -> Switch12/3
  MATLAB Function2/2(acc_b) -> MATLAB Function1/1(acc_b)
  MATLAB Function1/1(acc_g) -> Subsystem1/2(acc_g_filt)  "Am"
  Subsystem1/1(acc_moni) -> acc_moni/1
  track_deriv/1 -> Subsystem2/1(track_deriv)
  RC_in/1 -> Subsystem3/1(rc_in)
  Bus Selector9/1 -> Subsystem2/2(trk_deriv_sw), Subsystem/4(trk_deriv_sw)  "<G_TRK_DERIV>"

== system gnc_simplified/bus_generator ==
  guidance_out : Inport  OutDataTypeStr=Bus: IFRCG_Bus_GuidanceCmd
  Bus Creator : BusCreator  Inputs=8  OutDataTypeStr=Bus: IFRCG_Bus_Topic_TestSetpointsMonitor
      settings: InheritFromInputs=off
  Bus Selector : BusSelector  OutputSignals=trk_cmd,att_cmd
  Demux : Demux  Outputs=2
  Demux1 : Demux  Outputs=3
  Selector : Selector  InputPortWidth=3  IndexOptions=Index vector (dialog)  Indices=[1 3]  OutputSizes=1
  Selector1 : Selector  InputPortWidth=5  IndexOptions=Index vector (dialog)  Indices=[5 2 4]  OutputSizes=1
  codegen_topic_publication : Subsystem
  codegen_topic_subscription : Subsystem
  publish_topic : Constant  Value=true  OutDataTypeStr=boolean
  timestamp : Constant  Value=0  OutDataTypeStr=uint64
  test_setpoints : Outport  OutDataTypeStr=Bus: IFRCG_Bus_Topic_TestSetpointsMonitor
  wires:
  Demux1/3 -> Bus Creator/6
  Demux/2 -> Bus Creator/3
  Bus Creator/1 -> test_setpoints/1
  timestamp/1 -> Bus Creator/1
  Demux1/1 -> Bus Creator/4
  publish_topic/1 -> codegen_topic_publication/1(publish_topic)
  codegen_topic_publication/1(bus_codegen_topic_publication) -> Bus Creator/8
  codegen_topic_subscription/1(bus_codegen_topic_subscription) -> Bus Creator/7
  guidance_out/1 -> Bus Selector/1
  Demux1/2 -> Bus Creator/5
  Demux/1 -> Bus Creator/2
  Bus Selector/2 -> Selector1/1  "<att_cmd>"
  Bus Selector/1 -> Selector/1  "<trk_cmd>"
  Selector/1 -> Demux/1
  Selector1/1 -> Demux1/1

== system gnc_simplified/bus_generator1 ==
  ap_mde : Inport  OutDataTypeStr=uint8
  axis_modes : Inport  Port=2
  Bus Creator : BusCreator  Inputs=8  OutDataTypeStr=Bus: IFRCG_Bus_Topic_ApState
      settings: InheritFromInputs=off
  Data Type Conversion : DataTypeConversion  OutDataTypeStr=int32  SaturateOnIntegerOverflow=off  RndMeth=Floor
  Demux1 : Demux
  codegen_topic_publication : Subsystem
  codegen_topic_subscription : Subsystem
  publish_topic : Constant  Value=true  OutDataTypeStr=boolean
  timestamp : Constant  Value=0  OutDataTypeStr=uint64
  ap_modes : Outport  OutDataTypeStr=Bus: IFRCG_Bus_Topic_ApState
  wires:
  Demux1/1 -> Bus Creator/3
  Demux1/4 -> Bus Creator/6
  codegen_topic_subscription/1(bus_codegen_topic_subscription) -> Bus Creator/7
  codegen_topic_publication/1(bus_codegen_topic_publication) -> Bus Creator/8
  publish_topic/1 -> codegen_topic_publication/1(publish_topic)
  Demux1/3 -> Bus Creator/5
  timestamp/1 -> Bus Creator/1
  Bus Creator/1 -> ap_modes/1
  Demux1/2 -> Bus Creator/4
  ap_mde/1 -> Data Type Conversion/1
  Data Type Conversion/1 -> Bus Creator/2
  axis_modes/1 -> Demux1/1

== system gnc_simplified/INDI/Attitude ==
  note: alpha
      | theta
      | beta
      | psi
      | mu
  param : Inport  OutDataTypeStr=Bus: IFRCG_Bus_Params_Gnc
  att_direct : Inport  Port=2
  roll_lim : Inport  Port=3  OutDataTypeStr=single  PortDimensions=1
  d/dt_gachiv_m : Inport  Port=4  OutDataTypeStr=single  PortDimensions=3
  att_ctrl : Inport  Port=5
  gachi_m : Inport  Port=6
  att_m : Inport  Port=7
  axis_modes : Inport  Port=8
  MATLAB Function : MATLAB Function  TreatAsAtomicUnit=on
  Nonlinear_inversion : Subsystem
  Pseudo-control : Subsystem
  pqr_c : Outport
  att_moni : Outport  Port=2  OutDataTypeStr=single  PortDimensions=20
  wires:
  att_m/1 -> Pseudo-control/3(att_m), Nonlinear_inversion/3(att_m)
  param/1 -> Nonlinear_inversion/2(param), Pseudo-control/4(param)
  d/dt_gachiv_m/1 -> Nonlinear_inversion/4(d/dt_gachiv_m)
  gachi_m/1 -> Nonlinear_inversion/5(path_m)
  MATLAB Function/1(att_c) -> Pseudo-control/1(att_c)
  Nonlinear_inversion/1(rates_ltd) -> pqr_c/1
  Pseudo-control/2(d/dt_att_c) -> Nonlinear_inversion/1(d/dt_att_c)
  Pseudo-control/1(att_moni) -> att_moni/1
  roll_lim/1 -> Pseudo-control/2(roll_lim)
  axis_modes/1 -> MATLAB Function/3(modes)
  att_ctrl/1 -> MATLAB Function/2(guidance)
  att_direct/1 -> MATLAB Function/1(direct)

== system gnc_simplified/INDI/Monitor ==
  note: uint64 timestamp
      | float32[3] track_cmd
      | float32[3] track_m
      | float32[3] track_err
      | float32[3] gamma_dot_pid
      | float32[2] chi_dot_pd
      | float32[3] track_dot_cmd
      | float32[3] track_dot_m
      | float32[3] track_dot_err
      | float32[3] att_inc_cmd
      | float32[5] att_cmd
      | float32[5] att_m
      | float32[5] att_err
      | float32[5] att_dot_cmd
      | float32 delta_t
      | float32 t_m
      | float32 t_c
      | float32 chi_dot_cmd
      | float32 chi_dot_m
      | float32 chi_dot_err
      | float32 chi_ddot_cmd
      | float32[3] pqr_cmd
      | float32[3] pqr_m
      | float32[3] pqr_err
      | float32[3] pqr_dot_cmd
      | float32[3] pqr_dot_m
      | float32[3] pqr_dot_err
      | float32[3] delta_act
      | float32[3] act_m
      | float32[3] act_c
      | float32 nw_c
  note: float32[3] track_cmd
      | float32[3] track_m
      | float32[3] track_err
      | float32[3] gamma_dot_pid
      | float32[2] chi_dot_pd
      | float32[3] track_dot_cmd
      | float32[3] track_dot_m
      | float32[3] track_dot_err
      | float32[3] att_inc_cmd
  note: float32[5] att_cmd
      | float32[5] att_m
      | float32[5] att_err
      | float32[5] att_dot_cmd
  note: float32 delta_t
      | float32 t_m
      | float32 t_c
  note: float32 chi_dot_cmd
      | float32 chi_dot_m
      | float32 chi_dot_err
      | float32 chi_ddot_cmd
      | float32[3] pqr_cmd
      | float32[3] pqr_m
      | float32[3] pqr_err
      | float32[3] pqr_dot_cmd
      | float32[3] pqr_dot_m
      | float32[3] pqr_dot_err
      | float32[3] delta_act
      | float32[3] act_m
      | float32[3] act_c
      | float32 nw_c
  rte_moni : Inport  OutDataTypeStr=single  PortDimensions=32
  att_moni : Inport  Port=2  OutDataTypeStr=single  PortDimensions=20
  thr_moni : Inport  Port=3  OutDataTypeStr=single  PortDimensions=3
  path_moni : Inport  Port=4  OutDataTypeStr=single  PortDimensions=26
  Bus Creator1 : BusCreator  Inputs=33  OutDataTypeStr=Bus: IFRCG_Bus_Topic_IndiMonitor
      settings: InheritFromInputs=off
  Bus Selector1 : BusSelector  OutputSignals=signal1,signal2,signal3,signal4
  Bus Selector2 : BusSelector  OutputSignals=signal1.signal1,signal1.signal2,signal1.signal3,signal1.signal4,signal1.signal5,signal1.signal6,signal1.signal7,signal1.signal8,signal1.signal9,signal1.signal10,signal2.signal1,signal2.signal2,signal2.signal3,signal3
  Bus Selector3 : BusSelector  OutputSignals=signal1.signal1,signal1.signal2,signal1.signal3,signal1.signal4,signal1.signal5,signal1.signal6,signal1.signal7,signal1.signal8,att_inc_reciprocal
  Demux4 : Demux  Outputs=3
  codegen_topic_publication : Subsystem
  codegen_topic_subscription : Subsystem
  publish_topic : Constant  Value=true  OutDataTypeStr=boolean
  timestamp : Constant  Value=0  OutDataTypeStr=uint64
  indi_monitor : Outport  OutDataTypeStr=Bus: IFRCG_Bus_Topic_IndiMonitor
  wires:
  thr_moni/1 -> Demux4/1
  timestamp/1 -> Bus Creator1/1  "valid"
  Bus Creator1/1 -> indi_monitor/1
  Demux4/1 -> Bus Creator1/15
  Demux4/2 -> Bus Creator1/16
  Demux4/3 -> Bus Creator1/17
  Bus Selector2/1 -> Bus Creator1/18  "<signal1>"
  Bus Selector2/2 -> Bus Creator1/19  "<signal2>"
  Bus Selector2/3 -> Bus Creator1/20  "<signal3>"
  Bus Selector2/4 -> Bus Creator1/21  "<signal4>"
  Bus Selector2/5 -> Bus Creator1/22  "<signal5>"
  Bus Selector2/6 -> Bus Creator1/23  "<signal6>"
  Bus Selector2/8 -> Bus Creator1/25  "<signal8>"
  Bus Selector2/9 -> Bus Creator1/26  "<signal9>"
  Bus Selector2/10 -> Bus Creator1/27  "<signal10>"
  Bus Selector2/7 -> Bus Creator1/24  "<signal7>"
  Bus Selector2/14 -> Bus Creator1/31  "<signal3>"
  Bus Selector2/13 -> Bus Creator1/30  "<signal3>"
  Bus Selector2/11 -> Bus Creator1/28  "<signal1>"
  Bus Selector2/12 -> Bus Creator1/29  "<signal2>"
  Bus Selector3/1 -> Bus Creator1/2  "<signal1>"
  Bus Selector3/2 -> Bus Creator1/3  "<signal2>"
  Bus Selector3/3 -> Bus Creator1/4  "<signal3>"
  Bus Selector3/4 -> Bus Creator1/5  "<signal4>"
  Bus Selector3/5 -> Bus Creator1/6  "<signal5>"
  Bus Selector3/6 -> Bus Creator1/7  "<signal6>"
  Bus Selector3/7 -> Bus Creator1/8  "<signal7>"
  Bus Selector3/8 -> Bus Creator1/9  "<signal8>"
  Bus Selector1/1 -> Bus Creator1/11  "<signal1>"
  Bus Selector1/2 -> Bus Creator1/12  "<signal2>"
  Bus Selector1/3 -> Bus Creator1/13  "<signal3>"
  Bus Selector1/4 -> Bus Creator1/14  "<signal4>"
  path_moni/1 -> Bus Selector3/1
  att_moni/1 -> Bus Selector1/1
  rte_moni/1 -> Bus Selector2/1
  Bus Selector3/9 -> Bus Creator1/10  "<att_inc_reciprocal>"
  publish_topic/1 -> codegen_topic_publication/1(publish_topic)
  codegen_topic_subscription/1(bus_codegen_topic_subscription) -> Bus Creator1/32
  codegen_topic_publication/1(bus_codegen_topic_publication) -> Bus Creator1/33

== system gnc_simplified/INDI/Path ==
  note: [alpha,theta,beta,psi,mu]
  note: for attitude dynamics
  note: float32[3] track_cmd
      | float32[3] track_m
      | float32[3] track_err
      | float32[3] gamma_dot_pid
      | float32[2] chi_dot_pd
      | float32[3] track_dot_cmd
      | float32[3] track_dot_m
      | float32[3] track_dot_err
      | float32[3] att_inc_cmd
  gachiv_c : Inport  OutDataTypeStr=single  PortDimensions=3
  acc_k : Inport  Port=2
  Vk : Inport  Port=3  OutDataTypeStr=single  PortDimensions=1
  att_m : Inport  Port=4
  gachi_m : Inport  Port=5  OutDataTypeStr=single  PortDimensions=2
  track_deriv : Inport  Port=6
  params : Inport  Port=7  OutDataTypeStr=Bus: IFRCG_Bus_Params_Gnc
  q_dyn : Inport  Port=8
  Bus Creator : BusCreator  Inputs=2
  Incremental_inversion : Subsystem
  MATLAB Function : MATLAB Function  TreatAsAtomicUnit=on
  Mux1 : Mux  Inputs=2
  Mux3 : Mux  Inputs=2
  Pseudo-control : Subsystem
  Selector1 : Selector  InputPortWidth=5  IndexOptions=Index vector (dialog)  Indices=[1 3 5]  OutputSizes=1
  Selector2 : Selector  InputPortWidth=3  IndexOptions=Index vector (dialog)  Indices=3  OutputSizes=1
  Selector3 : Selector  InputPortWidth=5  IndexOptions=Index vector (dialog)  Indices=5  OutputSizes=1
  d/dt_gachiv_m : Outport  OutDataTypeStr=single  PortDimensions=3
  angles_c : Outport  Port=2  OutDataTypeStr=single  PortDimensions=5
  path_moni : Outport  Port=3
  thr_inc : Outport  Port=4  OutDataTypeStr=single  PortDimensions=1
  wires:
  Incremental_inversion/1(angles_c) -> angles_c/1
  att_m/1 -> Selector3/1, Selector1/1
  acc_k/1 -> MATLAB Function/1(acc_k)
  Pseudo-control/2(d/dt_gachiv_e) -> Incremental_inversion/1(d/dt_gachiv_e)
  Mux1/1 -> Incremental_inversion/3(gachiv_m), Pseudo-control/5(gachiv_m)
  gachi_m/1 -> Mux1/1
  Vk/1 -> Mux1/2, MATLAB Function/2(Vk)
  Selector1/1 -> Incremental_inversion/4(abmu_m)
  Selector3/1 -> Pseudo-control/4(phi_m)
  MATLAB Function/2(v_dot) -> Mux3/2
  Mux3/1 -> Pseudo-control/1(d/dt_gachiv_m), d/dt_gachiv_m/1
  params/1 -> Incremental_inversion/2(params), Pseudo-control/3(para)
  Incremental_inversion/2(inc_cmd) -> Bus Creator/2, Selector2/1
  q_dyn/1 -> Incremental_inversion/5(q_dyn)
  Pseudo-control/1(path_moni) -> Bus Creator/1
  track_deriv/1 -> Mux3/1
  Bus Creator/1 -> path_moni/1
  Selector2/1 -> thr_inc/1
  gachiv_c/1 -> Pseudo-control/2(gachiv_c)

== system gnc_simplified/INDI/Rates to surfaces&brakes ==
  note: float32 chi_dot_cmd
      | float32 chi_dot_m
      | float32 chi_dot_err
      | float32 chi_ddot_cmd
      | float32[3] pqr_cmd
      | float32[3] pqr_m
      | float32[3] pqr_err
      | float32[3] pqr_dot_cmd
      | float32[3] pqr_dot_m
      | float32[3] pqr_dot_err
      | float32[3] delta_act
      | float32[3] act_m
      | float32[3] act_c
      | float32 nw
  q_dyn : Inport
  rate_m : Inport  Port=2
  rate_ctrl : Inport  Port=3
  act_m : Inport  Port=4  OutDataTypeStr=single  PortDimensions=4
  params : Inport  Port=5  OutDataTypeStr=Bus: IFRCG_Bus_Params_Gnc
  inc_margins : Inport  Port=6  OutDataTypeStr=single  PortDimensions=[3,2]
  act_limits : Inport  Port=7
  imu_filter : Inport  Port=8
  Bus Creator : BusCreator  Inputs=3
  Constant : Constant  Value=0  OutDataTypeStr=single
  Demux : Demux  Outputs=3
  Diff and Filter IMU : Subsystem
      settings: PortSchema="{\"entries\":[{\"content\":{\"sides\":[{\"content\":{\"connectorIds\":[\"In1\",\"In2\",\"In3\"]},\"type\":\"ConnectorPlacement.EquallySpacedRectSide\",\"uuid\":\"595f2c85-6cd2-4ac4-94a6-147e3cdaf62c\"},{\"content\":{\"connectorIds\":[\"Out1\",\"Out2\"],\"side\":\"RIGHT\"},\"type\":\"ConnectorPlacement.EquallySpacedRectSide\",\"uuid\":\"fac480cf-7efe-4f97-8544-e0f640d96e89\"},{\"content\":{\"connectorIds\":[\"In4\"],\"side\":\"TOP\"},\"type\":\"ConnectorPlacement.EquallySpacedRectSide\",\"uuid\":\"db60b5ab-e407-476e-aa28-a63f2500fd6d\"}]},\"type\":\"ConnectorPlacement.EquallySpacedConnector\",\"uuid\":\"42848a63-649d-42c6-8a03-05f224ad5118\"}],\"packageUris\":[\"http://schema.mathworks.com/mf0/Connector/R2020b\"],\"version\":\"1.0\"}"
  Incremental_inversion : Subsystem
      settings: PortSchema="{\"entries\":[{\"content\":{\"sides\":[{\"content\":{\"connectorIds\":[\"In1\",\"In2\",\"In3\",\"In4\",\"In5\"]},\"type\":\"ConnectorPlacement.EquallySpacedRectSide\",\"uuid\":\"2477ed7f-2e4a-4d34-9191-aa6cd1598ace\"},{\"content\":{\"connectorIds\":[\"Out1\",\"Out2\",\"Out3\"],\"side\":\"RIGHT\"},\"type\":\"ConnectorPlacement.EquallySpacedRectSide\",\"uuid\":\"a67f6923-e928-4938-ab2a-8a1d443bfb45\"},{\"content\":{\"connectorIds\":[\"In6\"],\"side\":\"TOP\"},\"type\":\"ConnectorPlacement.EquallySpacedRectSide\",\"uuid\":\"ece43f97-e3a7-408a-af02-d9e4d3d20b00\"}]},\"type\":\"ConnectorPlacement.EquallySpacedConnector\",\"uuid\":\"8ca6f7dd-4284-4525-a7ce-c1aaa2c7f949\"}],\"packageUris\":[\"http://schema.mathworks.com/mf0/Connector/R2020b\"],\"version\":\"1.0\"}"
  Pseudo-control : Subsystem
      settings: PortSchema="{\"entries\":[{\"content\":{\"sides\":[{\"content\":{\"connectorIds\":[\"In1\",\"In2\",\"In3\"]},\"type\":\"ConnectorPlacement.EquallySpacedRectSide\",\"uuid\":\"2477ed7f-2e4a-4d34-9191-aa6cd1598ace\"},{\"content\":{\"connectorIds\":[\"Out1\",\"Out2\"],\"side\":\"RIGHT\"},\"type\":\"ConnectorPlacement.EquallySpacedRectSide\",\"uuid\":\"a67f6923-e928-4938-ab2a-8a1d443bfb45\"},{\"content\":{\"connectorIds\":[\"In4\"],\"side\":\"TOP\"},\"type\":\"ConnectorPlacement.EquallySpacedRectSide\",\"uuid\":\"ece43f97-e3a7-408a-af02-d9e4d3d20b00\"}]},\"type\":\"ConnectorPlacement.EquallySpacedConnector\",\"uuid\":\"8ca6f7dd-4284-4525-a7ce-c1aaa2c7f949\"}],\"packageUris\":[\"http://schema.mathworks.com/mf0/Connector/R2020b\"],\"version\":\"1.0\"}"
  Scope : Scope  NumInputPorts=3
      settings: ActiveDisplayYMinimum=-0.13287401574803148  ActiveDisplayYMaximum=0.13779527559055116  DataLoggingVariableName=ScopeData6
  control_surfaces : Outport  OutDataTypeStr=single  PortDimensions=3
  rte_moni : Outport  Port=2  OutDataTypeStr=single  PortDimensions=32
  inc_moni : Outport  Port=3
  wires:
  Incremental_inversion/1(act) -> control_surfaces/1, Demux/1
  Incremental_inversion/3(srfc_moni) -> Bus Creator/2
  Pseudo-control/2(rte_moni) -> Bus Creator/1
  params/1 -> Diff and Filter IMU/4(params), Pseudo-control/4(param), Incremental_inversion/6(params)
  rate_m/1 -> Diff and Filter IMU/3(rates), Pseudo-control/2(rate_m)
  Pseudo-control/1(d/dt_pqr_e) -> Incremental_inversion/5(d/dt_pqr_e)
  act_m/1 -> Diff and Filter IMU/2(act_m)
  Incremental_inversion/2(inc_moni) -> inc_moni/1
  Diff and Filter IMU/2(d/dt_pqr_m) -> Pseudo-control/1(pqr_dot_m)
  Bus Creator/1 -> rte_moni/1
  Demux/2 -> Scope/2  "ele_cmd"
  Demux/3 -> Scope/3  "rud_cmd"
  Demux/1 -> Scope/1  "ail_cmd"
  Diff and Filter IMU/1(act_del) -> Incremental_inversion/4(act_del)
  q_dyn/1 -> Incremental_inversion/3(q_dyn)
  inc_margins/1 -> Incremental_inversion/2(inc_margins)
  act_limits/1 -> Incremental_inversion/1(act_limits)
  imu_filter/1 -> Diff and Filter IMU/1(imu_filter)
  Constant/1 -> Bus Creator/3
  rate_ctrl/1 -> Pseudo-control/3(rte_c)
